simulink model "Basic_Controllers_Blocks"  (R2015b)
settings: Solver=ode45  StartTime=0.0  StopTime=100  FixedStep=0.1  RelTol=1e-3
values from neighbouring files (symbols this model uses):
  Jr = 6.06e-6    (= 6.06e-06)    [param.m]
  La = 0.0026    [param.m]
  N = 10000    [param.m]
  Ra = 3.647    [param.m]
  Tfv = 2.611e-6    (= 2.611e-06)    [param.m]
undefined symbols (not defined in the file or in its folder): kd, ke, ki, kp, kt, Vin
settings Model: Creator=catalin  LastModifiedBy=catalin

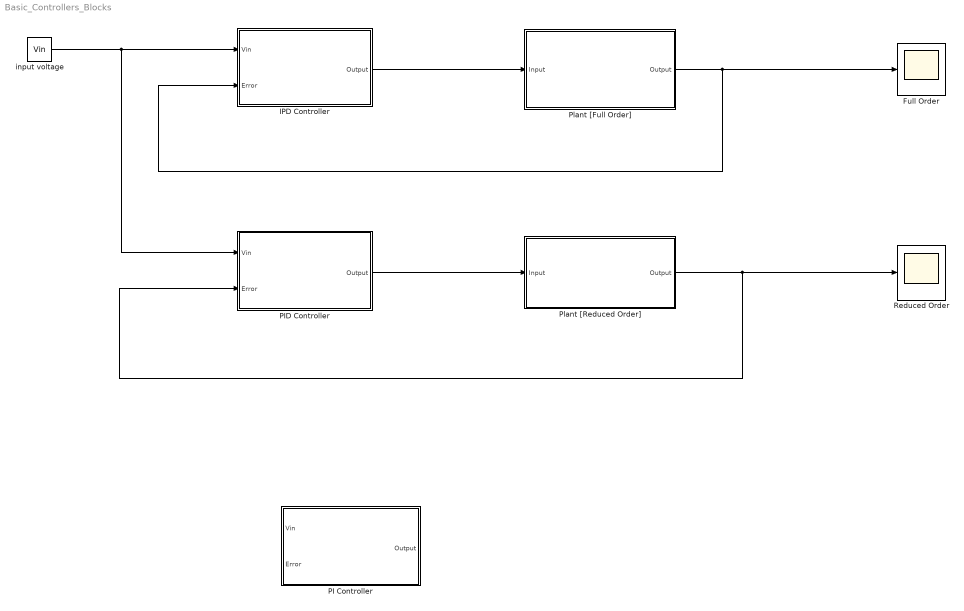
== system Basic_Controllers_Blocks ==
  Full Order : Scope
  IPD Controller : Subsystem
  PI Controller : Subsystem
  PID Controller : Subsystem
  Plant [Full Order] : Subsystem
  Plant [Reduced Order] : Subsystem
  Reduced Order : Scope
  input voltage : Constant  Value=Vin
  wires:
  input voltage/1 -> PID Controller/1(Vin), IPD Controller/1(Vin)
  IPD Controller/1(Output) -> Plant [Full Order]/1(Input)
  Plant [Reduced Order]/1(Output) -> PID Controller/2(Error), Reduced Order/1
  Plant [Full Order]/1(Output) -> IPD Controller/2(Error), Full Order/1
  PID Controller/1(Output) -> Plant [Reduced Order]/1(Input)

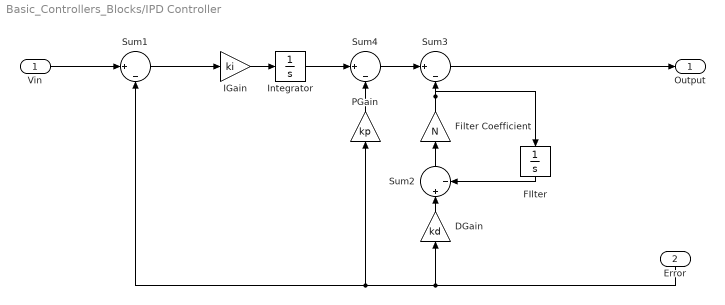
== system Basic_Controllers_Blocks/IPD Controller ==
  Vin : Inport
  Error : Inport  Port=2
  "DGain " : Gain  Gain=kd
  FIlter : Integrator
  Filter Coefficient : Gain  Gain=N
  IGain : Gain  Gain=ki
  Integrator : Integrator
  PGain : Gain  Gain=kp
  Sum{1..4} (4 alike) : Sum  Inputs=||+|-
  Output : Outport
  wires:
  FIlter/1 -> Sum2/2
  Sum4/1 -> Sum3/1
  Error/1 -> PGain/1, Sum1/2, "DGain "/1
  PGain/1 -> Sum4/2
  IGain/1 -> Integrator/1
  Vin/1 -> Sum1/1
  Integrator/1 -> Sum4/1
  Sum1/1 -> IGain/1
  Sum2/1 -> Filter Coefficient/1
  "DGain "/1 -> Sum2/1
  Filter Coefficient/1 -> FIlter/1, Sum3/2
  Sum3/1 -> Output/1

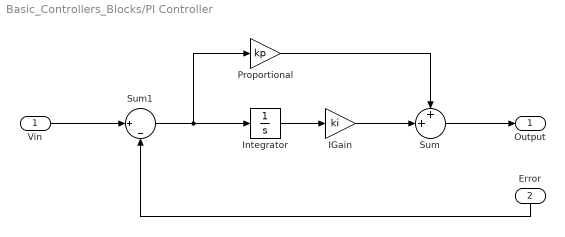
== system Basic_Controllers_Blocks/PI Controller ==
  Vin : Inport
  Error : Inport  Port=2
  IGain : Gain  Gain=ki
  Integrator : Integrator
  Proportional : Gain  Gain=kp
  Sum : Sum  Inputs=++|
  Sum1 : Sum  Inputs=||+|-
  Output : Outport
  wires:
  Error/1 -> Sum1/2
  Vin/1 -> Sum1/1
  Proportional/1 -> Sum/1
  Sum1/1 -> Integrator/1, Proportional/1
  Integrator/1 -> IGain/1
  IGain/1 -> Sum/2
  Sum/1 -> Output/1

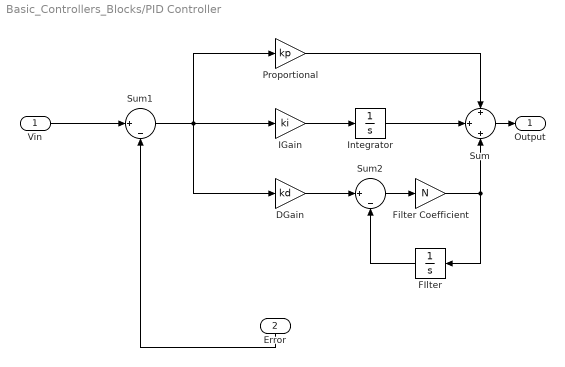
== system Basic_Controllers_Blocks/PID Controller ==
  Vin : Inport
  Error : Inport  Port=2
  "DGain " : Gain  Gain=kd
  FIlter : Integrator
  Filter Coefficient : Gain  Gain=N
  IGain : Gain  Gain=ki
  Integrator : Integrator
  Proportional : Gain  Gain=kp
  Sum : Sum  Inputs=+|+|+
  Sum1 : Sum  Inputs=||+|-
  Sum2 : Sum  Inputs=||+|-
  Output : Outport
  wires:
  Error/1 -> Sum1/2
  Vin/1 -> Sum1/1
  Proportional/1 -> Sum/1
  Sum1/1 -> IGain/1, "DGain "/1, Proportional/1
  Sum/1 -> Output/1
  "DGain "/1 -> Sum2/1
  Sum2/1 -> Filter Coefficient/1
  Filter Coefficient/1 -> Sum/3, FIlter/1
  FIlter/1 -> Sum2/2
  IGain/1 -> Integrator/1
  Integrator/1 -> Sum/2

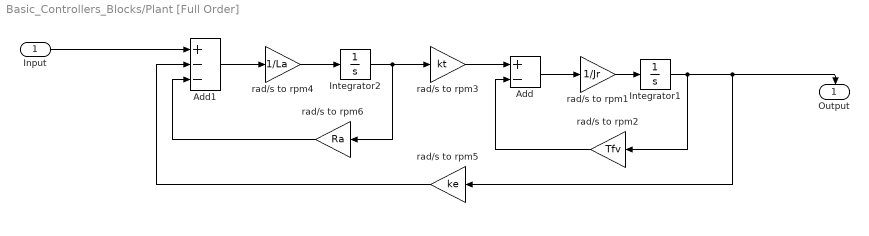
== system Basic_Controllers_Blocks/Plant [Full Order] ==
  Input : Inport
  Add : Sum  Inputs=+-
  Add1 : Sum  Inputs=+--
  Integrator1 : Integrator
  Integrator2 : Integrator
  rad/s to rpm1 : Gain  Gain=1/Jr
  rad/s to rpm2 : Gain  Gain=Tfv
  rad/s to rpm3 : Gain  Gain=kt
  rad/s to rpm4 : Gain  Gain=1/La
  rad/s to rpm5 : Gain  Gain=ke
  rad/s to rpm6 : Gain  Gain=Ra
  Output : Outport
  wires:
  Input/1 -> Add1/1
  rad/s to rpm1/1 -> Integrator1/1
  rad/s to rpm2/1 -> Add/2
  rad/s to rpm4/1 -> Integrator2/1
  rad/s to rpm3/1 -> Add/1
  rad/s to rpm5/1 -> Add1/2
  Integrator2/1 -> rad/s to rpm6/1, rad/s to rpm3/1
  Add1/1 -> rad/s to rpm4/1
  Add/1 -> rad/s to rpm1/1
  Integrator1/1 -> rad/s to rpm2/1, Output/1, rad/s to rpm5/1
  rad/s to rpm6/1 -> Add1/3

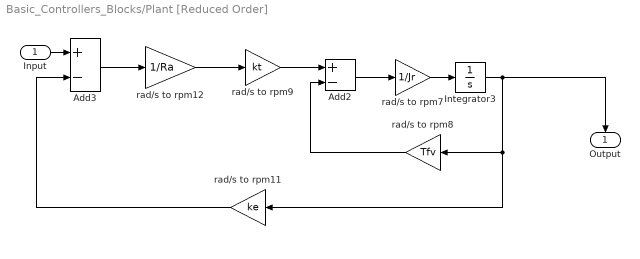
== system Basic_Controllers_Blocks/Plant [Reduced Order] ==
  Input : Inport
  Add2 : Sum  Inputs=+-
  Add3 : Sum  Inputs=+-
  Integrator3 : Integrator
  rad/s to rpm11 : Gain  Gain=ke
  rad/s to rpm12 : Gain  Gain=1/Ra
  rad/s to rpm7 : Gain  Gain=1/Jr
  rad/s to rpm8 : Gain  Gain=Tfv
  rad/s to rpm9 : Gain  Gain=kt
  Output : Outport
  wires:
  Add2/1 -> rad/s to rpm7/1
  Integrator3/1 -> Output/1, rad/s to rpm11/1, rad/s to rpm8/1
  rad/s to rpm12/1 -> rad/s to rpm9/1
  Input/1 -> Add3/1
  rad/s to rpm7/1 -> Integrator3/1
  rad/s to rpm11/1 -> Add3/2
  Add3/1 -> rad/s to rpm12/1
  rad/s to rpm9/1 -> Add2/1
  rad/s to rpm8/1 -> Add2/2
